simulink model "riggs"  (R2021a)
settings: Solver=VariableStepAuto  StartTime=0.0  StopTime=300.0  RelTol=1e-3
libraries: simulink x1
settings Model: Creator=Hansa Niluka  LastModifiedBy=Hansa Niluka

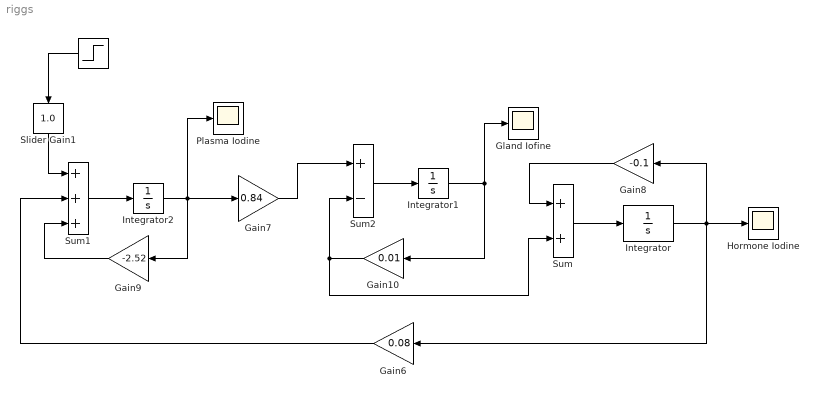
== system riggs ==
  " " : Step  Time=0  After=15  SampleTime=0
  Gain10 : Gain  Gain=0.01
  Gain6 : Gain  Gain=0.08
  Gain7 : Gain  Gain=0.84
  Gain8 : Gain  Gain=-0.1
  Gain9 : Gain  Gain=-2.52
  Gland Iofine : Scope
  Hormone Iodine : Scope
  Integrator : Integrator  InitialCondition=682
  Integrator1 : Integrator  InitialCondition=6821
  Integrator2 : Integrator  InitialCondition=81.2
  Plasma Iodine : Scope
  Slider Gain1 : simulink/Math Operations/Slider Gain  gain=1.0  low=0  high=2
  Sum : Sum
  Sum1 : Sum  Inputs=+++
  Sum2 : Sum  Inputs=+-
  wires:
  Sum1/1 -> Integrator2/1
  Slider Gain1/1 -> Sum1/1
  Gain6/1 -> Sum1/2
  " "/1 -> Slider Gain1/1
  Sum2/1 -> Integrator1/1
  Gain10/1 -> Sum2/2, Sum/2
  Gain9/1 -> Sum1/3
  Sum/1 -> Integrator/1
  Integrator2/1 -> Gain7/1, Plasma Iodine/1, Gain9/1
  Gain8/1 -> Sum/1
  Gain7/1 -> Sum2/1
  Integrator1/1 -> Gland Iofine/1, Gain10/1
  Integrator/1 -> Gain8/1, Hormone Iodine/1, Gain6/1
